simulink model "decoder"  (R2018b)
settings: Solver=FixedStepDiscrete  StartTime=0.0  StopTime=10.0  RelTol=1e-3
libraries: simulink x3, hdlsllib x2
settings Model: Creator=jayakumarav  LastModifiedBy=hiterd
settings DebuggingCC: LibraryContextMissingDiagnostic=none
settings SFSimCC: SimUseLocalCustomCode=off
settings RTWCC: RTWUseLocalCustomCode=off

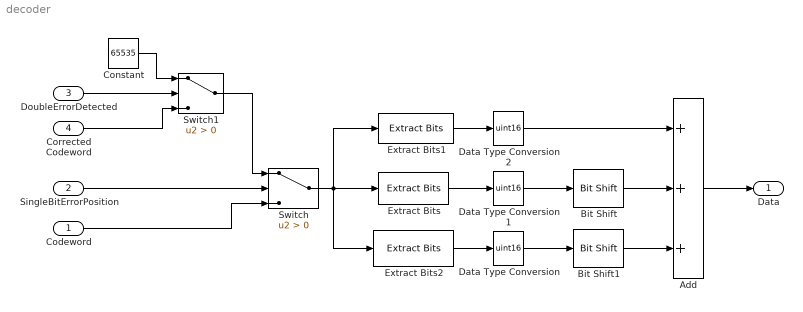
== system decoder ==
  Codeword : Inport
  SingleBitErrorPosition : Inport  Port=2  OutDataTypeStr=uint16
  DoubleErrorDetected : Inport  Port=3  OutDataTypeStr=boolean
  Corrected Codeword : Inport  Port=4
  Add : Sum  Inputs=+++
  Bit Shift : hdlsllib/Logic and Bit Operations/Bit Shift  mode=Shift Left Logical  N=1
      settings: SourceProductName=HDL Coder  SourceProductBaseCode=HD
  Bit Shift1 : hdlsllib/Logic and Bit Operations/Bit Shift  mode=Shift Left Logical  N=4
      settings: SourceProductName=HDL Coder  SourceProductBaseCode=HD
  Constant : Constant  Value=65535  OutDataTypeStr=uint16
  Data Type Conversion : DataTypeConversion  OutDataTypeStr=uint16
  Data Type Conversion1 : DataTypeConversion  OutDataTypeStr=uint16
  Data Type Conversion2 : DataTypeConversion  OutDataTypeStr=uint16
  Extract Bits : simulink/Logic and Bit Operations/Extract Bits  bitsToExtract=Range of bits  numBits=8  bitIdxRange=[5 7]  outScalingMode=Treat bit field as an integer
      settings: SourceProductName=Simulink
  Extract Bits1 : simulink/Logic and Bit Operations/Extract Bits  bitsToExtract=Range of bits  numBits=8  bitIdxRange=[3]  outScalingMode=Treat bit field as an integer
      settings: SourceProductName=Simulink
  Extract Bits2 : simulink/Logic and Bit Operations/Extract Bits  bitsToExtract=Range of bits  numBits=8  bitIdxRange=[9 15]  outScalingMode=Treat bit field as an integer
      settings: SourceProductName=Simulink
  Switch : Switch  Criteria=u2 > Threshold
  Switch1 : Switch  Criteria=u2 > Threshold
  Data : Outport
  wires:
  Corrected Codeword/1 -> Switch1/3
  DoubleErrorDetected/1 -> Switch1/2
  Switch1/1 -> Switch/1
  Constant/1 -> Switch1/1
  Extract Bits2/1 -> Data Type Conversion/1
  Switch/1 -> Extract Bits1/1, Extract Bits2/1, Extract Bits/1
  Codeword/1 -> Switch/3
  Extract Bits1/1 -> Data Type Conversion2/1
  Bit Shift/1 -> Add/2
  Add/1 -> Data/1
  Bit Shift1/1 -> Add/3
  SingleBitErrorPosition/1 -> Switch/2
  Data Type Conversion/1 -> Bit Shift1/1
  Data Type Conversion1/1 -> Bit Shift/1
  Extract Bits/1 -> Data Type Conversion1/1
  Data Type Conversion2/1 -> Add/1
